simulink library "csu_fpt_feature_point_lib"  (R2014b)
settings: Solver=ode45  SolverMode=SingleTasking  StartTime=0.0  StopTime=10.0  RelTol=1e-3
values from neighbouring files (symbols this model uses):
  cam_intrinsic_matrix_c = [ cam_focal_length_f/cam_pixel_size  0                                  cam_image_cx ... (first row only)    [csc_cam_camera_system_prep.m]
  fpt_ground_point = [0 0 0]    [csu_fpt_feature_point_init.m]
undefined symbols (not defined in the file or in its folder): ini_alt_wrt_1738rad
libraries: util_common_lib x2, util_frame_rotation_lib x1
settings Model: Creator=hcannon  LastModifiedBy=mstewart

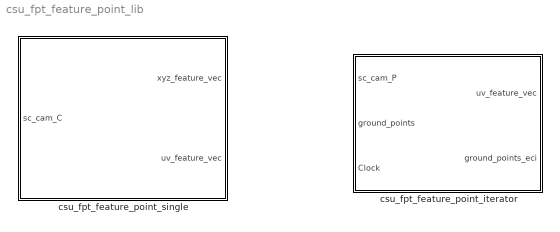
== system csu_fpt_feature_point_lib ==
  csu_fpt_feature_point_iterator : Subsystem  TreatAsAtomicUnit=on
  csu_fpt_feature_point_single : Subsystem

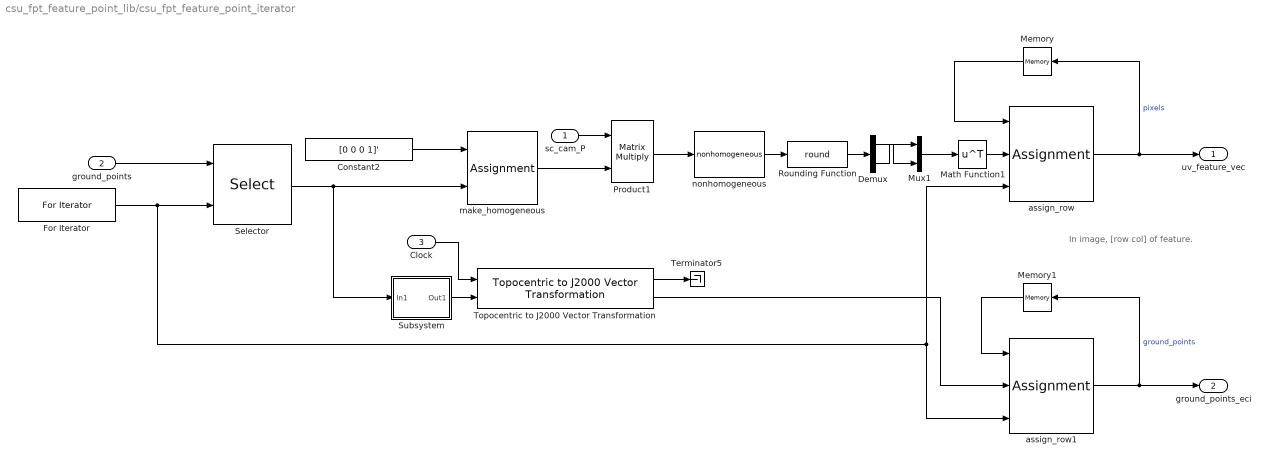
== system csu_fpt_feature_point_lib/csu_fpt_feature_point_iterator ==
  note: In image, [row col] of feature.
  sc_cam_P : Inport
  ground_points : Inport  Port=2
  "Clock " : Inport  Port=3
  Constant2 : Constant  Value=[0 0 0 1]'  VectorParams1D=off
  Demux : Demux  Outputs=2
  For Iterator : ForIterator  IterationLimit=15
  Math Function1 : Math  Operator=transpose  SaturateOnIntegerOverflow=on
  Memory : Memory  X0=zeros(15,2)  InheritSampleTime=on
  Memory1 : Memory  X0=zeros(15,3)  InheritSampleTime=on
  Mux1 : Mux  Inputs=2
  Product1 : Product  Multiplication=Matrix(*)  RndMeth=Zero
  Rounding Function : Rounding  Operator=round
  Selector : Selector  NumberOfDimensions=2  InputPortWidth=[10 2]  IndexOptions=Index vector (port),Select all  Indices=[1 3],1  OutputSizes=1,1
  Subsystem : Subsystem
  Terminator5 : Terminator
  "Topocentric to J2000 Vector Transformation " : util_frame_rotation_lib/Topocentric to J2000 Vector Transformation   SystemSampleTime=-1
  assign_row : Assignment  NumberOfDimensions=2  IndexOptions=Index vector (port),Assign all  Indices=1,1  OutputSizes=1,1
  assign_row1 : Assignment  NumberOfDimensions=2  IndexOptions=Index vector (port),Assign all  Indices=1,1  OutputSizes=1,1
  make_homogeneous : Assignment  Indices=[1 2 3]
  nonhomogeneous : util_common_lib/nonhomogeneous  SystemSampleTime=-1
  uv_feature_vec : Outport
  ground_points_eci : Outport  Port=2
  wires:
  "Topocentric to J2000 Vector Transformation "/1 -> Terminator5/1
  "Topocentric to J2000 Vector Transformation "/2 -> assign_row1/2
  "Clock "/1 -> "Topocentric to J2000 Vector Transformation "/1
  Subsystem/1(Out1) -> "Topocentric to J2000 Vector Transformation "/2
  Selector/1 -> Subsystem/1(In1), make_homogeneous/2
  Memory1/1 -> assign_row1/1
  assign_row1/1 -> ground_points_eci/1, Memory1/1  "ground_points"
  Demux/1 -> Mux1/2
  Demux/2 -> Mux1/1
  Mux1/1 -> Math Function1/1
  Rounding Function/1 -> Demux/1
  Math Function1/1 -> assign_row/2
  Constant2/1 -> make_homogeneous/1
  sc_cam_P/1 -> Product1/1
  make_homogeneous/1 -> Product1/2
  Product1/1 -> nonhomogeneous/1
  nonhomogeneous/1 -> Rounding Function/1
  ground_points/1 -> Selector/1
  For Iterator/1 -> assign_row1/3, assign_row/3, Selector/2
  assign_row/1 -> uv_feature_vec/1, Memory/1  "pixels"
  Memory/1 -> assign_row/1

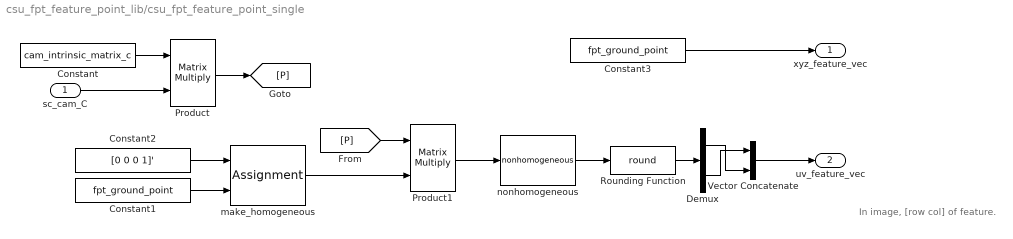
== system csu_fpt_feature_point_lib/csu_fpt_feature_point_single ==
  note: In image, [row col] of feature.
  sc_cam_C : Inport
  Constant : Constant  Value=cam_intrinsic_matrix_c
  Constant1 : Constant  Value=fpt_ground_point
  Constant2 : Constant  Value=[0 0 0 1]'
  Constant3 : Constant  Value=fpt_ground_point
  Demux : Demux  Outputs=2
  Product : Product  Multiplication=Matrix(*)  RndMeth=Zero
  Product1 : Product  Multiplication=Matrix(*)  RndMeth=Zero
  Rounding Function : Rounding  Operator=round
  Vector Concatenate : Concatenate
  make_homogeneous : Assignment  Indices=[1 2 3]
  nonhomogeneous : util_common_lib/nonhomogeneous  SystemSampleTime=-1
  xyz_feature_vec : Outport
  uv_feature_vec : Outport  Port=2
  wires:
  Vector Concatenate/1 -> uv_feature_vec/1
  Demux/1 -> Vector Concatenate/2
  Demux/2 -> Vector Concatenate/1
  Rounding Function/1 -> Demux/1
  Constant/1 -> Product/1
  sc_cam_C/1 -> Product/2
  Product/1 -> [P]
  Constant1/1 -> make_homogeneous/2
  Constant2/1 -> make_homogeneous/1
  [P] -> Product1/1
  make_homogeneous/1 -> Product1/2
  Product1/1 -> nonhomogeneous/1
  nonhomogeneous/1 -> Rounding Function/1
  Constant3/1 -> xyz_feature_vec/1

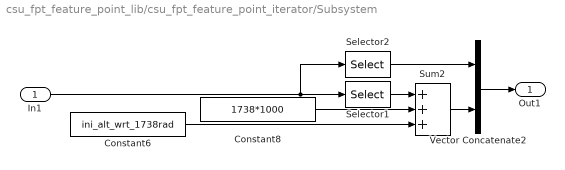
== system csu_fpt_feature_point_lib/csu_fpt_feature_point_iterator/Subsystem ==
  In1 : Inport
  Constant6 : Constant  Value=ini_alt_wrt_1738rad
  Constant8 : Constant  Value=1738*1000
  Selector1 : Selector  InputPortWidth=3  Indices=[3]
  Selector2 : Selector  InputPortWidth=3  Indices=[1 2]
  Sum2 : Sum  Inputs=+++
  Vector Concatenate2 : Concatenate
  Out1 : Outport
  wires:
  Vector Concatenate2/1 -> Out1/1
  Sum2/1 -> Vector Concatenate2/2
  Selector1/1 -> Sum2/1
  Selector2/1 -> Vector Concatenate2/1
  Constant8/1 -> Sum2/2
  Constant6/1 -> Sum2/3
  In1/1 -> Selector2/1, Selector1/1
